simulink model "ob_reg2"  (R2016b)
settings: Solver=FixedStepAuto  StartTime=0.0  StopTime=15  FixedStep=0.01  RelTol=1e-3
values from neighbouring files (symbols this model uses):
  A = [2  -4  -1; 4  -2  -1; -4  0  -1]    [matlab.mat]    (also in obserwator_stanu.m = [2 -4 -1)
  B = [0 0 -2]    [matlab.mat]    (also in obserwator_stanu.m = [0;0;-2])
  C = [1 0 0]    [matlab.mat]    (also in obserwator_stanu.m)
  D = 0    [matlab.mat]    (also in obserwator_stanu.m = [0])
  H = [11 -3.54166666667 12.9166666667]    [matlab.mat]    (also in obserwator_stanu.m = L')
  Ki = 205    [matlab.mat]    (also in obserwator_stanu.m = K1(1,4))
  KK = [-41.75 118.875 -10.5]    [matlab.mat]    (also in obserwator_stanu.m = K1(1,1:3))
  N = -3.25    [matlab.mat]    (also in obserwator_stanu.m = K*Nx+Nu)
undefined symbols (not defined in the file or in its folder): sigbuilder_block
settings Model: Creator=lenovo  LastModifiedBy=lenovo

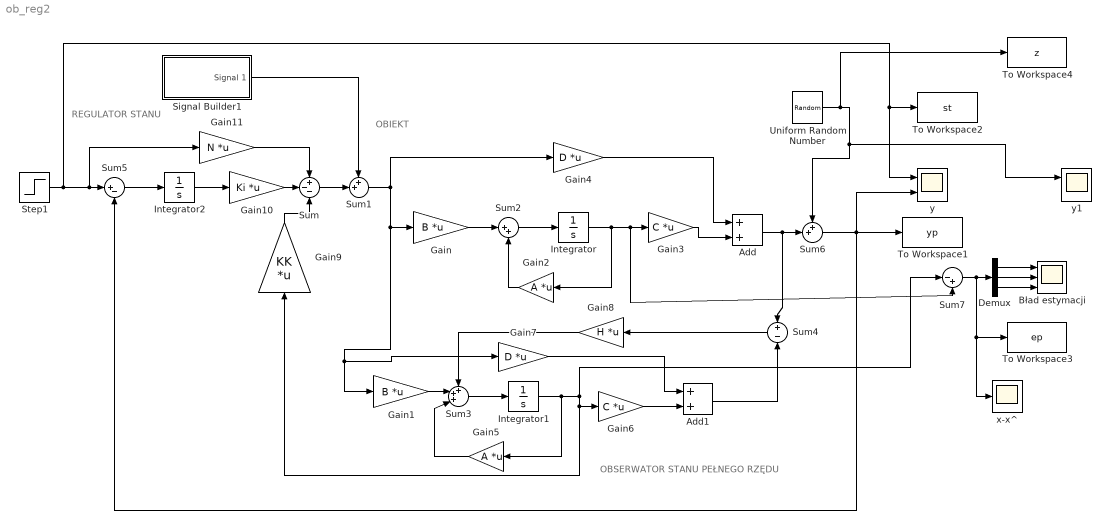
== system ob_reg2 ==
  note: OBSERWATOR STANU PEŁNEGO RZĘDU
  note: OBIEKT
  note: REGULATOR STANU
  Add : Sum
  Add1 : Sum
  Bład estymacji : Scope  NumInputPorts=3
  Demux : Demux  Outputs=3
  Gain : Gain  Gain=B  Multiplication=Matrix(K*u)
  Gain1 : Gain  Gain=B  Multiplication=Matrix(K*u)
  Gain10 : Gain  Gain=Ki  Multiplication=Matrix(K*u)
  Gain11 : Gain  Gain=N  Multiplication=Matrix(K*u)
  Gain2 : Gain  Gain=A  Multiplication=Matrix(K*u)
  Gain3 : Gain  Gain=C  Multiplication=Matrix(K*u)
  Gain4 : Gain  Gain=D  Multiplication=Matrix(K*u)
  Gain5 : Gain  Gain=A  Multiplication=Matrix(K*u)
  Gain6 : Gain  Gain=C  Multiplication=Matrix(K*u)
  Gain7 : Gain  Gain=D  Multiplication=Matrix(K*u)
  Gain8 : Gain  Gain=H  Multiplication=Matrix(K*u)
  Gain9 : Gain  Gain=KK  Multiplication=Matrix(K*u)
  Integrator : Integrator
  Integrator1 : Integrator
  Integrator2 : Integrator
  Signal Builder1 : Subsystem  Tag=STV Subsys  LoadFcn=sigbuilder_block('load');  StartFcn=sigbuilder_block('start');  StopFcn=sigbuilder_block('stop');  ClipboardFcn=sigbuilder_block('clipboard');  mask(Sigbuilder block){tuvar=[0:10]}
      mask help: Simulink:masks:SigbuilderBlock_MD
      mask init:
      | if ~strcmp(get_param(bdroot(gcbh),'SimulationStatus'),'stopped') tuvar = sigbuilder_block('maskInit'); end
      settings: CopyFcn=sigbuilder_block('copy');  DeleteFcn=sigbuilder_block('delete');  ModelCloseFcn=sigbuilder_block('modelClose');  PreSaveFcn=sigbuilder_block('preSave');  PauseFcn=sigbuilder_block('pause');  ContinueFcn=sigbuilder_block('continue');  NameChangeFcn=sigbuilder_block('namechange');  OpenFcn=sigbuilder_block('open',[437.25 153.75 550.5 359.25 ]);  CloseFcn=sigbuilder_block('close');
      mask Display: plot(0, 0, 100, 100,[2, 2, 32, 32, 2], [68, 8, 8, 68, 68],[32, 2], [38, 38], [32, 19, 2],[53, 60, 44], [32, 17, 17, 2],[16, 16, 31, 31]);txt = getActiveGroup(gcbh);text(2, 100, txt,'verticalAlignment', 'top');
  Step1 : Step  Time=0.1  SampleTime=0
  Sum : Sum  Inputs=+--
  Sum1 : Sum  Inputs=++|
  Sum2 : Sum  Inputs=|++
  Sum3 : Sum  Inputs=+++|
  Sum4 : Sum  Inputs=+|-
  Sum5 : Sum  Inputs=|+-
  Sum6 : Sum  Inputs=++|
  Sum7 : Sum  Inputs=|-+
  To Workspace1 : ToWorkspace  VariableName=yp  SaveFormat=Timeseries  SampleTime=-1
  To Workspace2 : ToWorkspace  VariableName=st  SaveFormat=Timeseries  SampleTime=-1
  To Workspace3 : ToWorkspace  VariableName=ep  SaveFormat=Timeseries  SampleTime=-1
  To Workspace4 : ToWorkspace  VariableName=z  SaveFormat=Timeseries  SampleTime=-1
  Uniform Random Number : UniformRandomNumber  Minimum=-0.01  Maximum=0.01  SampleTime=0.01
  x-x^ : Scope
  y : Scope  NumInputPorts=2
  y1 : Scope  NumInputPorts=2
  wires:
  Gain2/1 -> Sum2/2
  Gain/1 -> Sum2/1
  Sum2/1 -> Integrator/1
  Gain3/1 -> Add/2
  Gain4/1 -> Add/1
  Sum3/1 -> Integrator1/1
  Gain6/1 -> Add1/2
  Gain7/1 -> Add1/1
  Gain1/1 -> Sum3/2
  Gain5/1 -> Sum3/3
  Sum4/1 -> Gain8/1
  Gain8/1 -> Sum3/1
  Sum/1 -> Sum1/2
  Step1/1 -> To Workspace2/1, y/1, Gain11/1, Sum5/1
  Sum5/1 -> Integrator2/1
  Gain10/1 -> Sum/2
  Gain11/1 -> Sum/1
  Add/1 -> Sum6/2, Sum4/1
  Gain9/1 -> Sum/3
  Signal Builder1/1(Signal 1) -> Sum1/1
  Sum1/1 -> Gain7/1, Gain1/1, Gain/1, Gain4/1
  Integrator2/1 -> Gain10/1
  Add1/1 -> Sum4/2
  Uniform Random Number/1 -> To Workspace4/1, y1/1, Sum6/1
  Sum6/1 -> To Workspace1/1, y/2, Sum5/2
  Integrator/1 -> Gain2/1, Sum7/2, Gain3/1
  Integrator1/1 -> Gain5/1, Gain6/1, Gain9/1, Sum7/1
  Demux/1 -> Bład estymacji/1
  Demux/2 -> Bład estymacji/2
  Demux/3 -> Bład estymacji/3
  Sum7/1 -> To Workspace3/1, x-x^/1, Demux/1

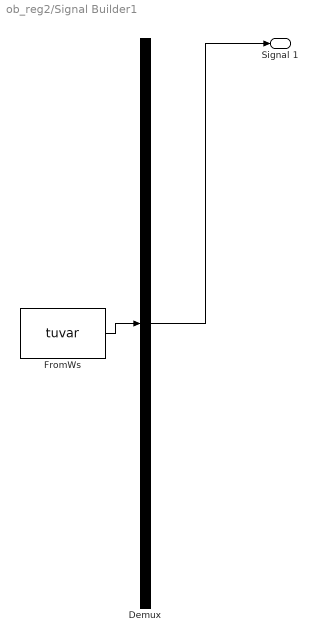
== system ob_reg2/Signal Builder1 ==
  Demux : Demux  Tag=STV Demux  Outputs=1
  FromWs : FromWorkspace  Tag=STV FromWs  VariableName=tuvar  SampleTime=0
      SigBuilderData=|
      | common.afterFinalStr = 'Extrapolate'
      | common.sampleTime = 0
      | dataSet.timeRange = [0 10]
      | dataSet.name = 'Group 1'
      | sbobj.Groups.Name = 'Group 1'
      | sbobj.Groups.Signals.Name = 'Signal 1'
      | sbobj.Groups.Signals.XData = [0 6 6 7.46 7.46 10]
      | sbobj.Groups.Signals.YData = [0 0 1.005 1.005 0 0]
  Signal 1 : Outport  Tag=STV Outport
  wires:
  Demux/1 -> Signal 1/1
  FromWs/1 -> Demux/1
